simulink model "SuspensionSystem"  (R2025a)
settings: Solver=ode45  StartTime=0.0  StopTime=500  MaxStep=1e-4  RelTol=1e-3
undefined symbols (not defined in the file): robot, susp, world
settings Model: Creator=yaremadzulynsky  LastModifiedBy=yaremadzulynsky

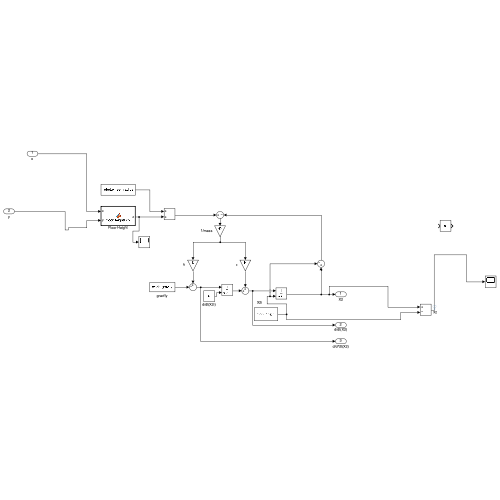
[thumbnail: Simulink's stored preview of the top-level diagram]
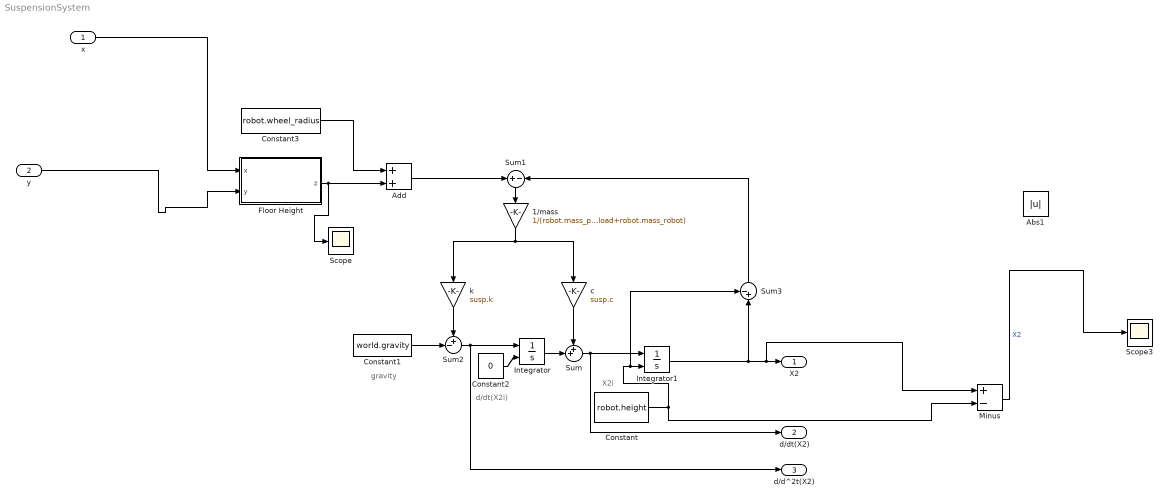
== system SuspensionSystem ==
  note: gravity
  note: X2i
  note: d/dt(X2i)
  x : Inport
  y : Inport  Port=2
  1/mass : Gain  Gain=1/(robot.mass_payload+robot.mass_robot)
  Abs1 : Abs  SaturateOnIntegerOverflow=off
  Add : Sum
  Constant : Constant  Value=robot.height
  Constant1 : Constant  Value=world.gravity
  Constant2 : Constant  Value=0
  Constant3 : Constant  Value=robot.wheel_radius
  Floor Height : MATLAB Function  TreatAsAtomicUnit=on
  Integrator : Integrator  InitialConditionSource=external
  Integrator1 : Integrator  InitialConditionSource=external
  Minus : Sum  Inputs=+-
  Scope : Scope
      settings: ActiveDisplayYMinimum=-0.020637943005678838  ActiveDisplayYMaximum=0.01666356223336515
  Scope3 : Scope
      settings: ActiveDisplayYMinimum=-0.018874999862712457  ActiveDisplayYMaximum=0.16987499876441214  DataLoggingVariableName=ScopeData3
  Sum : Sum  Inputs=++|
  Sum1 : Sum  Inputs=+-
  Sum2 : Sum  Inputs=+-|
  Sum3 : Sum  Inputs=-+|
  c : Gain  Gain=susp.c
  k : Gain  Gain=susp.k
  X2 : Outport
  d/dt(X2) : Outport  Port=2
  d/d^2t(X2) : Outport  Port=3
  wires:
  Integrator/1 -> Sum/2
  Sum2/1 -> d/d^2t(X2)/1, Integrator/1
  Constant1/1 -> Sum2/2
  Integrator1/1 -> Sum3/2, Minus/1, X2/1
  Sum1/1 -> 1/mass/1
  Sum/1 -> d/dt(X2)/1, Integrator1/1
  Constant2/1 -> Integrator/2
  c/1 -> Sum/1
  k/1 -> Sum2/1
  Constant/1 -> Sum3/1, Integrator1/2, Minus/2
  1/mass/1 -> k/1, c/1
  Sum3/1 -> Sum1/2
  Floor Height/1(z) -> Scope/1, Add/2
  Add/1 -> Sum1/1
  Constant3/1 -> Add/1
  x/1 -> Floor Height/1(x)
  y/1 -> Floor Height/2(y)
  Minus/1 -> Scope3/1  "X2"

== matlab function SuspensionSystem/Floor Height ==
  data: x input; z output; y input
function z = floorHeightFcn(x, y)
%#codegen
% FLOORHEIGHTFCN  Return floor height [m] at position (x,y).
% Suitable for MATLAB Function blocks (no dynamic sizing / cat / zeros).

%% ---- CONSTANTS --------------------------------------------------------
tile_pitch          = 0.3048;  % 1 ft in m
grout_width         = 0.010;   % 1 cm in m 
grout_depth         = 0.005;   % 5 mm in m
tile_surface_height = 0.0;     % set tile height to be our datum

threshold_start_x   = -1.0;    % x coordinate of door bump
threshold_length_x  = 0.05;    % bump length 5 cm in m
threshold_height    = 0.03;    % bump height 3 cm in m
threshold_y_min     = -0.5;    % doorway span in y
threshold_y_max     =  0.5;
%% -----------------------------------------------------------------------

%% ---- TILE + GROUT -----------------------------------------------------
% local coordinates inside a tile
x_mod = mod(x + tile_pitch/2, tile_pitch);
y_mod = mod(y + tile_pitch/2, tile_pitch);

% distance to nearest grout line in each axis
x_dist = min(x_mod, tile_pitch - x_mod);
y_dist = min(y_mod, tile_pitch - y_mod);

% haversine–shaped grout dips
tolerance = 5e-4;
gDipX = 0.0;
if x_dist < (grout_width/2 + tolerance)
    gDipX = grout_depth/2 * (1 + cos(2*pi*x_dist/grout_width));
end

gDipY = 0.0;
if y_dist < (grout_width/2 + tolerance)
    gDipY = grout_depth/2 * (1 + cos(2*pi*y_dist/grout_width));
end

% grout_valley = max(gDipX, gDipY);          % cross‑shaped groove
grout_valley = max(gDipX, gDipY);
z_tiles      = tile_surface_height - grout_valley;   % dips negative

%% ---- DOOR THRESHOLD bump ----------------------------------------------
if  threshold_height > 0    && ...
    x >= threshold_start_x  && x <= threshold_start_x + threshold_length_x && ...
    y >= threshold_y_min    && y <= threshold_y_max

    s_local = x - threshold_start_x;       % 0 → L
    z_bump  = threshold_height/2 * ...
              (1 - cos(2*pi*s_local/threshold_length_x));   % full‑cycle haversine
    z = tile_surface_height + z_bump;      % bump sits on flat tile
else
    z = z_tiles;                           % normal tile + grout
end
end
